simulink model "SVPWM"  (R2023a)
settings: Solver=FixedStepAuto  StartTime=0.0  StopTime=10.0  FixedStep=1e-6  RelTol=1e-3
values from neighbouring files (symbols this model uses):
  m = 0.71822373487189439    [SVPWM.sldd]
  TS = 0.0005    [SVPWM.sldd]
  Vdc = 750.0    [SVPWM.sldd]
libraries: spsSeriesRLCBranchLib x10, spsDCVoltageSourceLib x1, slpidlib x1, spsThreePhaseVIMeasurementLib x1, spsUniversalBridgeLib x1, sps_lib x1, spsabctoAlphaBetaZeroLib x1, simulink x1
settings Model: DataDictionary=SVPWM.sldd  SimulationMode=accelerator  Creator=86159  LastModifiedBy=86159

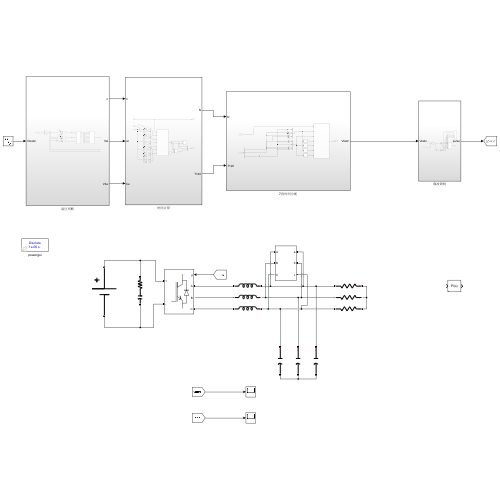
[thumbnail: Simulink's stored preview of the top-level diagram]
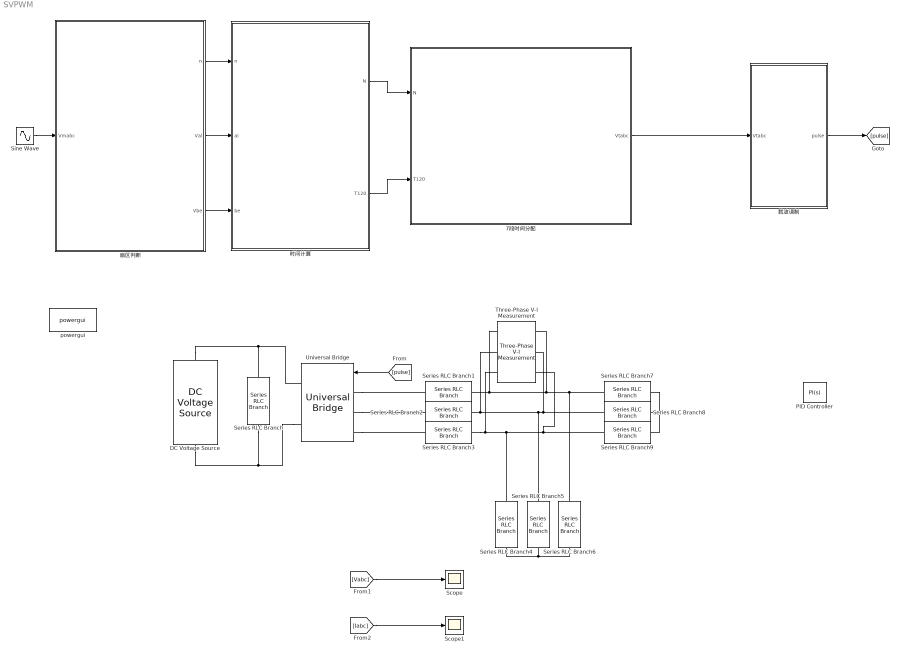
== system SVPWM ==
  7段时间分配 : Subsystem
  DC Voltage Source : spsDCVoltageSourceLib/DC Voltage Source  Amplitude=Vdc  Measurements=None
  PID Controller : slpidlib/PID Controller  Controller=PI  Form=Parallel  TimeDomain=Continuous-time  UseExternalTs=off  SampleTime=-1  IntegratorMethod=Forward Euler  FilterMethod=Forward Euler  ControllerParametersSource=internal  P=1  I=1  UseKiTs=off  D=0  N=100  UseFilter=on  TunerSelectOption=Transfer Function Based (PID Tuner App)  InitialConditionSource=internal  InitialConditionForIntegrator=0  InitialConditionForFilter=0  DifferentiatorICPrevScaledInput=0  ExternalReset=none  TrackingMode=off  Kt=1  LimitOutput=off  SatLimitsSource=internal  UpperSaturationLimit=inf  LowerSaturationLimit=-inf  LinearizeAsGain=on  AntiWindupMode=none  Kb=1  LimitIntegrator=off  UpperIntegratorSaturationLimit=inf  LowerIntegratorSaturationLimit=-inf  POutMin=[]  POutMax=[]  IOutMin=[]  IOutMax=[]  DOutMin=[]  DOutMax=[]  NOutMin=[]  NOutMax=[]  SumOutMin=[]  SumOutMax=[]  SaturationOutMin=[]  SaturationOutMax=[]  PParamMin=[]  PParamMax=[]  IParamMin=[]  IParamMax=[]  DParamMin=[]  DParamMax=[]  NParamMin=[]  NParamMax=[]  KbParamMin=[]  KbParamMax=[]  KtParamMin=[]  KtParamMax=[]  KbOutMin=[]  KbOutMax=[]  KtOutMin=[]  KtOutMax=[]  IntegratorOutMin=[]  IntegratorOutMax=[]  FilterOutMin=[]  FilterOutMax=[]  SumI1OutMin=[]  SumI1OutMax=[]  SumI2OutMin=[]  SumI2OutMax=[]  SumI3OutMin=[]  SumI3OutMax=[]  SumI4OutMin=[]  SumI4OutMax=[]  SumDOutMin=[]  SumDOutMax=[]  DifferentiatorOutMin=[]  DifferentiatorOutMax=[]  FilterDiffOutCoefMin=[]  FilterDiffOutCoefMax=[]  ReciprocalOutMin=[]  ReciprocalOutMax=[]  SumDenOutMin=[]  SumDenOutMax=[]  SumNumOutMin=[]  SumNumOutMax=[]  DivideOutMin=[]  DivideOutMax=[]  UdiffTsProdOutMin=[]  UdiffTsProdOutMax=[]  NTsProdOutMin=[]  NTsProdOutMax=[]  UintegralTsProdOutMin=[]  UintegralTsProdOutMax=[]  UngainTsProdOutMin=[]  UngainTsProdOutMax=[]  ClampingZeroOutDataTypeStr=Inherit: Inherit via back propagation  ClampingZeroOutMin=[]  ClampingZeroOutMax=[]  FilterDenConstantOutDataTypeStr=Inherit: Inherit via back propagation  FilterDenConstantOutMin=[]  FilterDenConstantOutMax=[]  PCopyOutDataTypeStr=Inherit: Inherit via back propagation  PCopyOutMin=[]  PCopyOutMax=[]  NCopyOutDataTypeStr=Inherit: Inherit via back propagation  NCopyOutMin=[]  NCopyOutMax=[]  IntegratorContinuousStateAttributes=''  IntegratorStateMustResolveToSignalObject=off  IntegratorRTWStateStorageClass=Auto  FilterContinuousStateAttributes=''  FilterStateMustResolveToSignalObject=off  FilterRTWStateStorageClass=Auto  ParallelPVariant=InternalParameters  IdealPVariant=Disabled  IVariant=InternalParameters  DVariant=Disabled  IntegratorVariant=Continuous  SatVariant=Disabled  AWVariant=Passthrough  PCopyVariant=Disabled  TRVariant=Disabled  FdbkBlocksVariant=Forward  IdealPFdbkVariant=Disabled  SatFdbkVariant=Disabled  DerivativeFilterVariant=Disabled  NVariant=Disabled  NCopyVariant=Disabled_SignalSpec  FilterICVariant=Disabled  IntegratorICVariant=InternalICs  ExternalResetVariant=Disabled  TRSumVariant=Passthrough  SumFdbkVariant=Disabled  SumVariant=Sum_PI  TsampFilterVariant=InternalTs  TsampNgainVariant=Passthrough  TsampIntegralVariant=Disabled_SignalSpec  ExternalSaturationOutDataTypeStr=Inherit: Same as second input
  Scope : Scope
  Scope1 : Scope
  Series RLC Branch : spsSeriesRLCBranchLib/Series RLC Branch  LConnTagsString=__new0  RConnTagsString=__new0  BranchType=RC  Resistance=1e-6  Inductance=1e-3  SetiL0=off  InitialCurrent=0  Capacitance=4000e-6  Setx0=off  InitialVoltage=0  Measurements=None
  Series RLC Branch1 : spsSeriesRLCBranchLib/Series RLC Branch  LConnTagsString=__new0  RConnTagsString=__new0  BranchType=L  Resistance=1  Inductance=6e-3  SetiL0=off  InitialCurrent=0  Capacitance=4000e-6  Setx0=off  InitialVoltage=0  Measurements=None
  Series RLC Branch2 : spsSeriesRLCBranchLib/Series RLC Branch  LConnTagsString=__new0  RConnTagsString=__new0  BranchType=L  Resistance=1  Inductance=6e-3  SetiL0=off  InitialCurrent=0  Capacitance=4000e-6  Setx0=off  InitialVoltage=0  Measurements=None
  Series RLC Branch3 : spsSeriesRLCBranchLib/Series RLC Branch  LConnTagsString=__new0  RConnTagsString=__new0  BranchType=L  Resistance=1  Inductance=6e-3  SetiL0=off  InitialCurrent=0  Capacitance=4000e-6  Setx0=off  InitialVoltage=0  Measurements=None
  Series RLC Branch4 : spsSeriesRLCBranchLib/Series RLC Branch  LConnTagsString=__new0  RConnTagsString=__new0  BranchType=C  Resistance=1  Inductance=6e-3  SetiL0=off  InitialCurrent=0  Capacitance=30e-6  Setx0=off  InitialVoltage=0  Measurements=None
  Series RLC Branch5 : spsSeriesRLCBranchLib/Series RLC Branch  LConnTagsString=__new0  RConnTagsString=__new0  BranchType=C  Resistance=1  Inductance=6e-3  SetiL0=off  InitialCurrent=0  Capacitance=30e-6  Setx0=off  InitialVoltage=0  Measurements=None
  Series RLC Branch6 : spsSeriesRLCBranchLib/Series RLC Branch  LConnTagsString=__new0  RConnTagsString=__new0  BranchType=C  Resistance=1  Inductance=6e-3  SetiL0=off  InitialCurrent=0  Capacitance=30e-6  Setx0=off  InitialVoltage=0  Measurements=None
  Series RLC Branch7 : spsSeriesRLCBranchLib/Series RLC Branch  LConnTagsString=__new0  RConnTagsString=__new0  BranchType=R  Resistance=10  Inductance=6e-3  SetiL0=off  InitialCurrent=0  Capacitance=4000e-6  Setx0=off  InitialVoltage=0  Measurements=None
  Series RLC Branch8 : spsSeriesRLCBranchLib/Series RLC Branch  LConnTagsString=__new0  RConnTagsString=__new0  BranchType=R  Resistance=10  Inductance=6e-3  SetiL0=off  InitialCurrent=0  Capacitance=4000e-6  Setx0=off  InitialVoltage=0  Measurements=None
  Series RLC Branch9 : spsSeriesRLCBranchLib/Series RLC Branch  LConnTagsString=__new0  RConnTagsString=__new0  BranchType=R  Resistance=10  Inductance=6e-3  SetiL0=off  InitialCurrent=0  Capacitance=4000e-6  Setx0=off  InitialVoltage=0  Measurements=None
  Sine Wave : Sin  Amplitude=m  Frequency=2*pi*50  Phase=[0 -2*pi/3 2*pi/3]  SampleTime=0
  Three-Phase V-I Measurement : spsThreePhaseVIMeasurementLib/Three-Phase V-I Measurement  VoltageMeasurement=phase-to-phase  SetLabelV=on  LabelV=Vabc  Vpu=off  VpuLL=off  CurrentMeasurement=yes  SetLabelI=on  LabelI=Iabc  Ipu=off  Pbase=100e6  Vbase=500e3  OutputType=Complex  PhasorSimulation=off  PSBequivalent=0
  Universal Bridge : spsUniversalBridgeLib/Universal Bridge  Arms=3  SnubberResistance=1e5  SnubberCapacitance=inf  Device=IGBT / Diodes  Ron=1e-3  Lon=0  ForwardVoltages="[  0  0  ]"  ForwardVoltage=0  GTOparameters=[ 10e-6 , 20e-6 ]  IGBTparameters=[ 1e-6 , 2e-6 ]  Measurements=None  Measurements_2=None  converterType=Rectifier
  powergui : sps_lib/powergui  Priority=1  SimulationMode=Discrete  SampleTime=1e-6  frequency=60  Iterations=50  frequencyindice=0  Pbase=100e6  ErrMax=1e-4  UnitsV=kV  UnitsW=MW  buscounter=0  FunctionMessages=off  echomessages=off  EnableUseOfTLC=off  CurrentSourceSwitches=off  DisableSnubberDevices=off  DisableRonSwitches=off  DisableVfSwitches=off  DisplayEquations=off  AutomaticDiscreteSolvers=off  SolverType=Tustin/Backward Euler (TBE)  Interpol=off  ExternalGateDelay=off  methode=off  Ts=100  x0status=blocks  SPID=on  SwTol=0  HookPort=off  NonlinearTolerance=1e-4  nMaxIteration=100  ContinueOnMaxIteration=off  RestoreLinks=warning  ResistiveCurrentMeasurement=off  Frange=[0:2:500]  Ylog=off  Xlog=on  ShowGrid=off  save=off  variable=ZData  structure=0  ZoomFFT=off  StartTime=0.0  cycles=1  DisplayStyle=1  fundamental=60  FreqAxis=off  MaxFrequency=1000  frequencyindicesteady=1  RmsSteady=1  display=off
  扇区判断 : Subsystem
  时间计算 : Subsystem
  载波调制 : Subsystem
  wires:
  扇区判断/1(n) -> 时间计算/1(n)
  Sine Wave/1 -> 扇区判断/1(Vmabc)
  扇区判断/2(Val) -> 时间计算/2(al)
  扇区判断/3(Vbe) -> 时间计算/3(be)
  时间计算/1(N) -> 7段时间分配/1(N)
  时间计算/2(T120) -> 7段时间分配/2(T120)
  7段时间分配/1(Vtabc) -> 载波调制/1(Vtabc)
  载波调制/1(pulse) -> [pulse]
  [pulse] -> Universal Bridge/1
  [Vabc] -> Scope/1
  [Iabc] -> Scope1/1
  connections:
  Universal Bridge/RConn2 -- DC Voltage Source/LConn1 -- Series RLC Branch/RConn1
  DC Voltage Source/RConn1 -- Universal Bridge/RConn1 -- Series RLC Branch/LConn1
  Universal Bridge/LConn1 -- Series RLC Branch1/RConn1
  Universal Bridge/LConn2 -- Series RLC Branch2/RConn1
  Universal Bridge/LConn3 -- Series RLC Branch3/RConn1
  Series RLC Branch3/LConn1 -- Three-Phase V-I Measurement/RConn3 -- Series RLC Branch9/RConn1 -- Series RLC Branch4/LConn1 -- Three-Phase V-I Measurement/LConn3
  Series RLC Branch2/LConn1 -- Three-Phase V-I Measurement/RConn2 -- Series RLC Branch8/RConn1 -- Series RLC Branch5/LConn1 -- Three-Phase V-I Measurement/LConn2
  Series RLC Branch1/LConn1 -- Three-Phase V-I Measurement/LConn1 -- Three-Phase V-I Measurement/RConn1 -- Series RLC Branch7/RConn1 -- Series RLC Branch6/LConn1
  Series RLC Branch5/RConn1 -- Series RLC Branch6/RConn1 -- Series RLC Branch4/RConn1
  Series RLC Branch7/LConn1 -- Series RLC Branch9/LConn1 -- Series RLC Branch8/LConn1

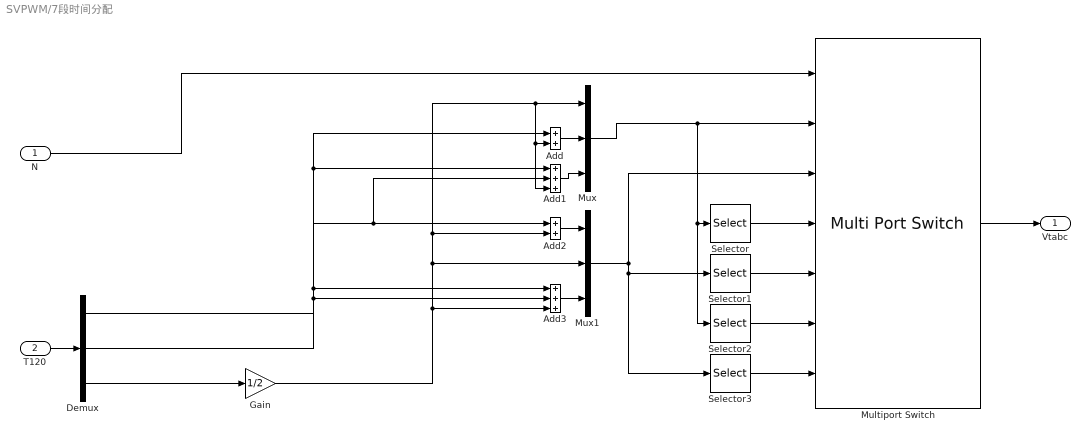
== system SVPWM/7段时间分配 ==
  N : Inport
  T120 : Inport  Port=2
  Add : Sum
  Add1 : Sum  Inputs=+++
  Add2 : Sum
  Add3 : Sum  Inputs=+++
  Demux : Demux  Outputs=3
  Gain : Gain  Gain=1/2
  Multiport Switch : MultiPortSwitch  Inputs=6  SaturateOnIntegerOverflow=off  InputSameDT=off
  Mux : Mux  Inputs=3
  Mux1 : Mux  Inputs=3
  Selector : Selector  InputPortWidth=3  IndexOptions=Index vector (dialog)  Indices=[3 1 2]  OutputSizes=1
  Selector1 : Selector  InputPortWidth=3  IndexOptions=Index vector (dialog)  Indices=[3 1 2]  OutputSizes=1
  Selector2 : Selector  InputPortWidth=3  IndexOptions=Index vector (dialog)  Indices=[2 3 1]  OutputSizes=1
  Selector3 : Selector  InputPortWidth=3  IndexOptions=Index vector (dialog)  Indices=[2 3 1]  OutputSizes=1
  Vtabc : Outport
  wires:
  Gain/1 -> Add3/3, Mux1/2, Add2/2, Add/2, Add1/3, Mux/1
  Add2/1 -> Mux1/1
  Selector2/1 -> Multiport Switch/6
  Mux/1 -> Selector2/1, Selector/1, Multiport Switch/2
  Demux/1 -> Add1/1, Add/1, Add3/1
  Mux1/1 -> Selector1/1, Selector3/1, Multiport Switch/3
  Demux/2 -> Add2/1, Add1/2, Add3/2
  Multiport Switch/1 -> Vtabc/1
  Add1/1 -> Mux/3
  Selector3/1 -> Multiport Switch/7
  Add3/1 -> Mux1/3
  Demux/3 -> Gain/1
  Add/1 -> Mux/2
  Selector/1 -> Multiport Switch/4
  Selector1/1 -> Multiport Switch/5
  T120/1 -> Demux/1
  N/1 -> Multiport Switch/1

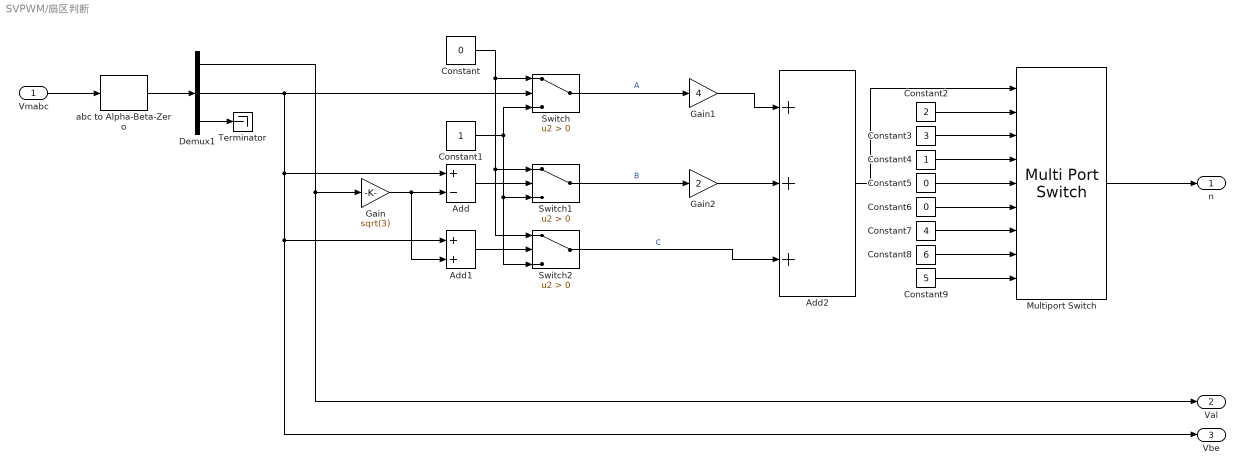
== system SVPWM/扇区判断 ==
  Vmabc : Inport
  Add : Sum  Inputs=+-
  Add1 : Sum
  Add2 : Sum  Inputs=+++
  Constant : Constant  Value=0
  Constant1 : Constant
  Constant2 : Constant  Value=2
  Constant3 : Constant  Value=3
  Constant4 : Constant
  Constant5 : Constant  Value=0
  Constant6 : Constant  Value=0
  Constant7 : Constant  Value=4
  Constant8 : Constant  Value=6
  Constant9 : Constant  Value=5
  Demux1 : Demux  Outputs=3
  Gain : Gain  Gain=sqrt(3)
  Gain1 : Gain  Gain=4
  Gain2 : Gain  Gain=2
  Multiport Switch : MultiPortSwitch  DataPortOrder=Zero-based contiguous  Inputs=8  zeroidx=on  SaturateOnIntegerOverflow=off  InputSameDT=off
  Switch : Switch  Criteria=u2 > Threshold  SaturateOnIntegerOverflow=off  InputSameDT=off
  Switch1 : Switch  Criteria=u2 > Threshold  SaturateOnIntegerOverflow=off  InputSameDT=off
  Switch2 : Switch  Criteria=u2 > Threshold  SaturateOnIntegerOverflow=off  InputSameDT=off
  Terminator : Terminator
  abc to Alpha-Beta-Zero : spsabctoAlphaBetaZeroLib/abc to Alpha-Beta-Zero
  n : Outport
  Val : Outport  Port=2
  Vbe : Outport  Port=3
  wires:
  Demux1/2 -> Switch/2, Add1/1, Vbe/1, Add/1
  Demux1/3 -> Terminator/1
  Vmabc/1 -> abc to Alpha-Beta-Zero/1
  Switch1/1 -> Gain2/1  "B"
  Constant1/1 -> Switch2/3, Switch1/3, Switch/3
  Constant7/1 -> Multiport Switch/7
  Gain2/1 -> Add2/2
  Gain/1 -> Add1/2, Add/2
  Constant5/1 -> Multiport Switch/5
  Constant/1 -> Switch1/1, Switch2/1, Switch/1
  abc to Alpha-Beta-Zero/1 -> Demux1/1
  Demux1/1 -> Val/1, Gain/1
  Constant9/1 -> Multiport Switch/9
  Constant6/1 -> Multiport Switch/6
  Constant8/1 -> Multiport Switch/8
  Switch/1 -> Gain1/1  "A"
  Add/1 -> Switch1/2
  Switch2/1 -> Add2/3  "C"
  Add2/1 -> Multiport Switch/1
  Add1/1 -> Switch2/2
  Gain1/1 -> Add2/1
  Constant2/1 -> Multiport Switch/2
  Constant4/1 -> Multiport Switch/4
  Constant3/1 -> Multiport Switch/3
  Multiport Switch/1 -> n/1

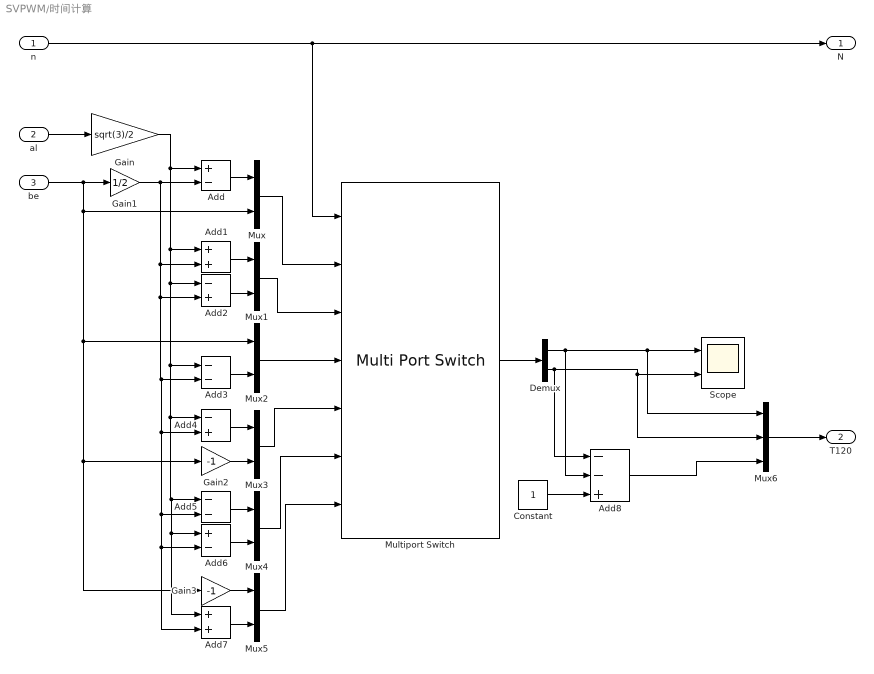
== system SVPWM/时间计算 ==
  n : Inport
  al : Inport  Port=2
  be : Inport  Port=3
  Add : Sum  Inputs=+-
  Add1 : Sum
  Add2 : Sum  Inputs=-+
  Add3 : Sum  Inputs=--
  Add4 : Sum  Inputs=-+
  Add5 : Sum  Inputs=--
  Add6 : Sum  Inputs=+-
  Add7 : Sum
  Add8 : Sum  Inputs=--+
  Constant : Constant
  Demux : Demux  Outputs=2
  Gain : Gain  Gain=sqrt(3)/2
  Gain1 : Gain  Gain=1/2
  Gain2 : Gain  Gain=-1
  Gain3 : Gain  Gain=-1
  Multiport Switch : MultiPortSwitch  Inputs=6  SaturateOnIntegerOverflow=off  InputSameDT=off
  Mux{,1..5} (6 alike) : Mux  Inputs=2
  Mux6 : Mux  Inputs=3
  Scope : Scope  NumInputPorts=2
  N : Outport
  T120 : Outport  Port=2
  wires:
  Demux/2 -> Add8/1, Mux6/2, Scope/2
  Mux/1 -> Multiport Switch/2
  Add5/1 -> Mux4/1
  be/1 -> Mux2/1, Gain3/1, Gain2/1, Mux/2, Gain1/1
  Gain/1 -> Add/1, Add7/1, Add6/1, Add5/1, Add4/1, Add3/1, Add2/1, Add1/1
  Add7/1 -> Mux5/2
  Mux5/1 -> Multiport Switch/7
  Multiport Switch/1 -> Demux/1
  Gain1/1 -> Add7/2, Add6/2, Add5/2, Add4/2, Add3/2, Add2/2, Add1/2, Add/2
  Mux4/1 -> Multiport Switch/6
  Mux2/1 -> Multiport Switch/4
  Add/1 -> Mux/1
  Add1/1 -> Mux1/1
  Add3/1 -> Mux2/2
  Gain2/1 -> Mux3/2
  Demux/1 -> Add8/2, Mux6/1, Scope/1
  Mux1/1 -> Multiport Switch/3
  Add6/1 -> Mux4/2
  Add4/1 -> Mux3/1
  Gain3/1 -> Mux5/1
  Add2/1 -> Mux1/2
  Add8/1 -> Mux6/3
  Mux3/1 -> Multiport Switch/5
  n/1 -> N/1, Multiport Switch/1
  Constant/1 -> Add8/3
  Mux6/1 -> T120/1
  al/1 -> Gain/1

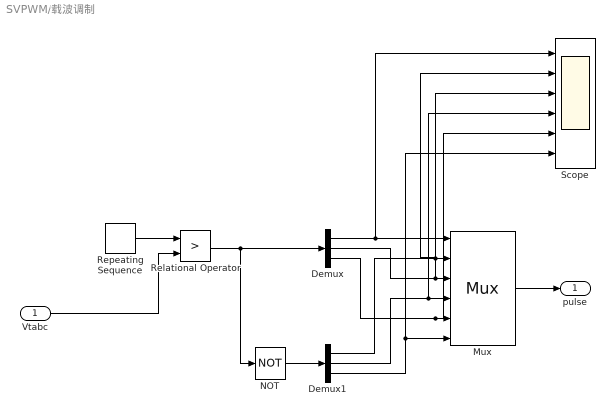
== system SVPWM/载波调制 ==
  Vtabc : Inport
  Demux : Demux  Outputs=3
  Demux1 : Demux  Outputs=3
  Mux : Mux  Inputs=6
  NOT : Logic  Operator=NOT  IconShape=distinctive  AllPortsSameDT=off  OutDataTypeStr=boolean
  Relational Operator : RelationalOperator  Operator=>  OutDataTypeStr=boolean  RndMeth=Simplest  InputSameDT=off
  Repeating Sequence : simulink/Sources/Repeating Sequence  rep_seq_t=[0 TS/2 TS]  rep_seq_y=[0 1 0]
  Scope : Scope  NumInputPorts=6
  pulse : Outport
  wires:
  Demux/1 -> Mux/1, Scope/1
  Relational Operator/1 -> NOT/1, Demux/1
  Demux1/1 -> Scope/2, Mux/2
  Repeating Sequence/1 -> Relational Operator/1
  Demux/3 -> Scope/5, Mux/5
  Demux/2 -> Scope/3, Mux/3
  NOT/1 -> Demux1/1
  Demux1/2 -> Mux/4, Scope/4
  Demux1/3 -> Mux/6, Scope/6
  Mux/1 -> pulse/1
  Vtabc/1 -> Relational Operator/2
